simulink model "BallAndPlate_AMPC_Controller"  (R2024b)
settings: configuration reference "controller_config_MPC" (kept outside this file)
undefined symbols (not defined in the file): BallAndPlate_ss_d, TimeStep_MPC, V_refNum
libraries: mpclib x1, sharedTrackingLibrary x1
settings Model: DataDictionary=BallAndPlate_system_data.sldd  Creator=tshintai  LastModifiedBy=tshintai
settings ConfigSetRef: SourceName=controller_config_MPC

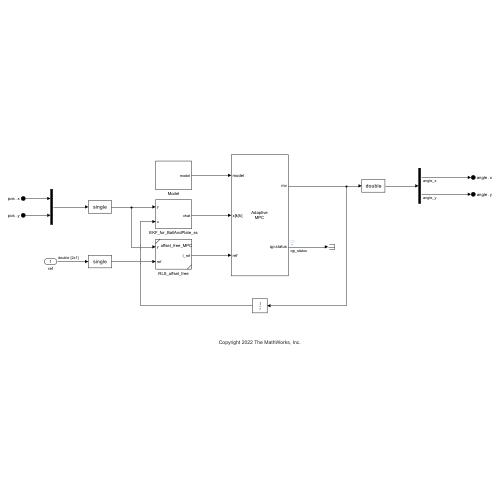
[thumbnail: Simulink's stored preview of the top-level diagram]
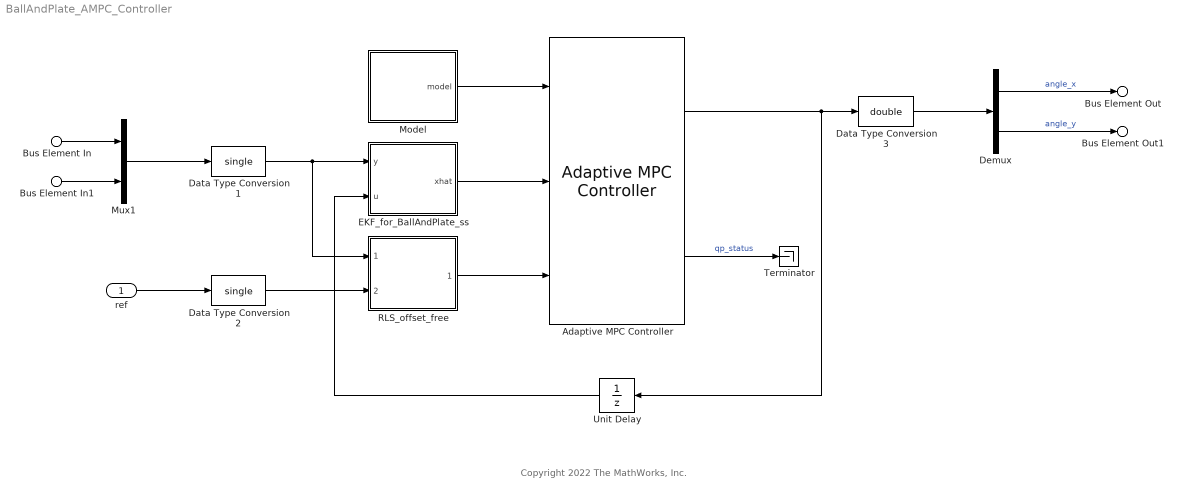
== system BallAndPlate_AMPC_Controller ==
  note: Copyright 2022 The MathWorks, Inc.
  ref : Inport  OutDataTypeStr=double  PortDimensions=[2, V_refNum]
  Bus Element In : Inport  Port=2  PortName=pos  Element=x
  Bus Element In1 : Inport  Port=2  PortName=pos  Element=y
  Adaptive MPC Controller : mpclib/Adaptive MPC Controller  SCDEnableBlockLinearizationSpecification=on  mpcobj=mpcObj  enable_value=0  updateMPCinCallerWorkspace=on  md_inport=off  mv_inport=off  uref_inport=off  return_cost=off  return_mvseq=off  return_qpstatus=on  return_xseq=off  return_state=off  return_ovseq=off  state_inport=on  isltv_plant=off  umin_inport=off  umax_inport=off  ymin_inport=off  ymax_inport=off  cc_inport=off  ywt_inport=off  uwt_inport=off  duwt_inport=off  rhoeps_inport=off  pm_inport=off  MaximumP=10  HorizonChoice=FixedHorizon  BlockDataType=single  SampleTimeInherited=off  switch_inport=off
  Data Type Conversion1 : DataTypeConversion  OutDataTypeStr=single  SaturateOnIntegerOverflow=off  RndMeth=Floor
  Data Type Conversion2 : DataTypeConversion  OutDataTypeStr=single  SaturateOnIntegerOverflow=off  RndMeth=Floor
  Data Type Conversion3 : DataTypeConversion  OutDataTypeStr=double  SaturateOnIntegerOverflow=off  RndMeth=Floor
  Demux : Demux  Outputs=2
  EKF_for_BallAndPlate_ss : Subsystem
  Model : Subsystem
  Mux1 : Mux  Inputs=2
  RLS_offset_free : Subsystem  ReferencedSubsystem=offset_free_MPC
  Terminator : Terminator
  Unit Delay : UnitDelay  SampleTime=-1  HasFrameUpgradeWarning=on
  Bus Element Out : Outport  PortName=angle  Element=x
  Bus Element Out1 : Outport  PortName=angle  Element=y
  wires:
  Bus Element In/1 -> Mux1/1
  Bus Element In1/1 -> Mux1/2
  Adaptive MPC Controller/2 -> Terminator/1  "qp_status"
  Data Type Conversion2/1 -> RLS_offset_free/2
  Model/1(model) -> Adaptive MPC Controller/1
  Adaptive MPC Controller/1 -> Data Type Conversion3/1, Unit Delay/1
  EKF_for_BallAndPlate_ss/1(xhat) -> Adaptive MPC Controller/2
  Unit Delay/1 -> EKF_for_BallAndPlate_ss/2(u)
  Data Type Conversion1/1 -> RLS_offset_free/1, EKF_for_BallAndPlate_ss/1(y)
  Data Type Conversion3/1 -> Demux/1
  Mux1/1 -> Data Type Conversion1/1
  Demux/1 -> Bus Element Out/1  "angle_x"
  Demux/2 -> Bus Element Out1/1  "angle_y"
  ref/1 -> Data Type Conversion2/1
  RLS_offset_free/1 -> Adaptive MPC Controller/3

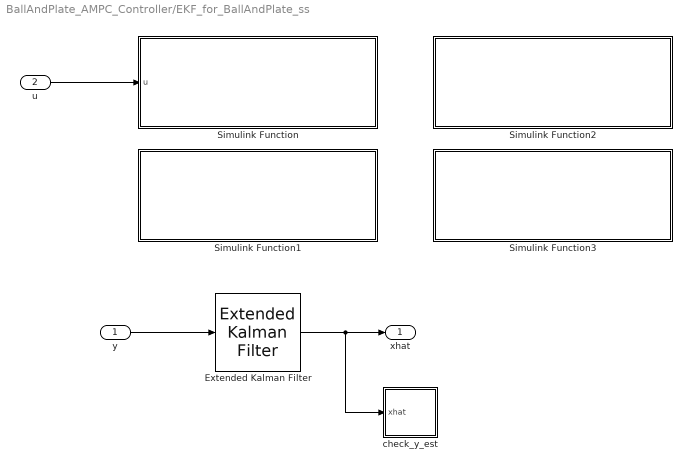
== system BallAndPlate_AMPC_Controller/EKF_for_BallAndPlate_ss ==
  y : Inport
  u : Inport  Port=2
  Extended Kalman Filter : sharedTrackingLibrary/Extended Kalman Filter  StateTransitionFcn=EKF_BAP_State_function  HasStateTransitionJacobianFcn=on  StateTransitionJacobianFcn=EKF_BAP_State_Jacobian  HasAdditiveProcessNoise=Additive  ProcessNoise=EKF_Q  HasTimeVaryingProcessNoise=off  HasStateTransitionFcnExtraArgument=0  InitialState=EKF_x_init  InitialStateCovariance=EKF_P_init  MeasurementFcn1=EKF_BAP_Measurement_function  HasMeasurementJacobianFcn1=on  MeasurementJacobianFcn1=EKF_BAP_Measurement_Jacobian  HasMeasurementEnablePort1=off  HasAdditiveMeasurementNoise1=Additive  MeasurementNoise1=EKF_R  HasTimeVaryingMeasurementNoise1=off  HasMeasurementFcnExtraArgument1=0  HasMeasurementWrapping1=off  MeasurementFcn2=myMeasurementFcn  HasMeasurementJacobianFcn2=off  HasMeasurementEnablePort2=off  HasAdditiveMeasurementNoise2=Additive  MeasurementNoise2=1  HasTimeVaryingMeasurementNoise2=off  HasMeasurementFcnExtraArgument2=0  HasMeasurementWrapping2=off  MeasurementFcn3=myMeasurementFcn  HasMeasurementJacobianFcn3=off  HasMeasurementEnablePort3=off  HasAdditiveMeasurementNoise3=Additive  MeasurementNoise3=1  HasTimeVaryingMeasurementNoise3=off  HasMeasurementFcnExtraArgument3=0  HasMeasurementWrapping3=off  MeasurementFcn4=myMeasurementFcn  HasMeasurementJacobianFcn4=off  HasMeasurementEnablePort4=off  HasAdditiveMeasurementNoise4=Additive  MeasurementNoise4=1  HasTimeVaryingMeasurementNoise4=off  HasMeasurementFcnExtraArgument4=0  HasMeasurementWrapping4=off  MeasurementFcn5=myMeasurementFcn  HasMeasurementJacobianFcn5=off  HasMeasurementEnablePort5=off  HasAdditiveMeasurementNoise5=Additive  MeasurementNoise5=1  HasTimeVaryingMeasurementNoise5=off  HasMeasurementFcnExtraArgument5=0  HasMeasurementWrapping5=off  EnableMultirate=off  StateTransitionFcnSampleTime=1  MeasurementFcn1SampleTime=1  MeasurementFcn2SampleTime=1  MeasurementFcn3SampleTime=1  MeasurementFcn4SampleTime=1  MeasurementFcn5SampleTime=1  UseCurrentEstimator=on  OutputStateCovariance=off  DataType=single  SampleTime=TimeStep_MPC  NumberOfMeasurements=1
  Simulink Function : Subsystem  TreatAsAtomicUnit=on
  Simulink Function1 : Subsystem  TreatAsAtomicUnit=on
  Simulink Function2 : Subsystem  TreatAsAtomicUnit=on
  Simulink Function3 : Subsystem  TreatAsAtomicUnit=on
  check_y_est : Subsystem
  xhat : Outport
  wires:
  u/1 -> Simulink Function/1(u)
  Extended Kalman Filter/1 -> check_y_est/1(xhat), xhat/1
  y/1 -> Extended Kalman Filter/1

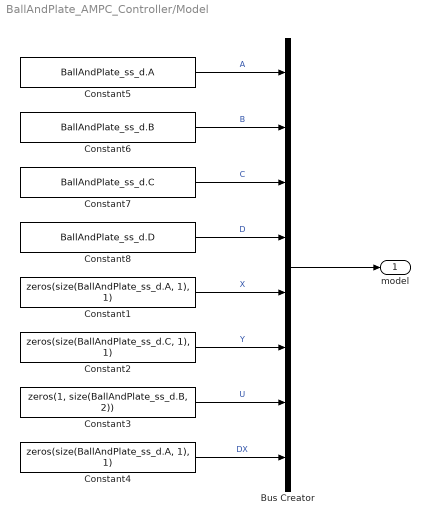
== system BallAndPlate_AMPC_Controller/Model ==
  Bus Creator : BusCreator  Inputs=8
  Constant1 : Constant  Value=zeros(size(BallAndPlate_ss_d.A, 1), 1)  VectorParams1D=off  OutDataTypeStr=single
  Constant2 : Constant  Value=zeros(size(BallAndPlate_ss_d.C, 1), 1)  VectorParams1D=off  OutDataTypeStr=single
  Constant3 : Constant  Value=zeros(1, size(BallAndPlate_ss_d.B, 2))  VectorParams1D=off  OutDataTypeStr=single
  Constant4 : Constant  Value=zeros(size(BallAndPlate_ss_d.A, 1), 1)  VectorParams1D=off  OutDataTypeStr=single
  Constant5 : Constant  Value=BallAndPlate_ss_d.A  VectorParams1D=off  OutDataTypeStr=single
  Constant6 : Constant  Value=BallAndPlate_ss_d.B  VectorParams1D=off  OutDataTypeStr=single
  Constant7 : Constant  Value=BallAndPlate_ss_d.C  VectorParams1D=off  OutDataTypeStr=single
  Constant8 : Constant  Value=BallAndPlate_ss_d.D  VectorParams1D=off  OutDataTypeStr=single
  model : Outport
  wires:
  Constant2/1 -> Bus Creator/6  "Y"
  Constant5/1 -> Bus Creator/1  "A"
  Constant6/1 -> Bus Creator/2  "B"
  Bus Creator/1 -> model/1
  Constant7/1 -> Bus Creator/3  "C"
  Constant8/1 -> Bus Creator/4  "D"
  Constant3/1 -> Bus Creator/7  "U"
  Constant4/1 -> Bus Creator/8  "DX"
  Constant1/1 -> Bus Creator/5  "X"

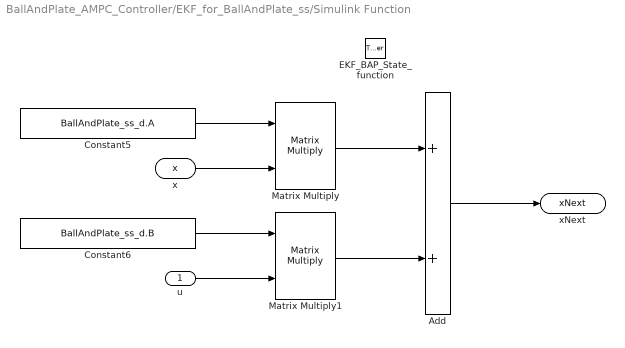
== system BallAndPlate_AMPC_Controller/EKF_for_BallAndPlate_ss/Simulink Function ==
  u : Inport
  EKF_BAP_State_function : TriggerPort  TriggerType=function-call  IsSimulinkFunction=on  FunctionName=EKF_BAP_State_function  FunctionVisibility=scoped  VariantControl=(inherit)
  Add : Sum
  Constant5 : Constant  Value=BallAndPlate_ss_d.A  VectorParams1D=off  OutDataTypeStr=single
  Constant6 : Constant  Value=BallAndPlate_ss_d.B  VectorParams1D=off  OutDataTypeStr=single
  Matrix Multiply : Product  Multiplication=Matrix(*)
  Matrix Multiply1 : Product  Multiplication=Matrix(*)
  x : ArgIn  DisableCoverage=on  OutDataTypeStr=single  PortDimensions=size(BallAndPlate_ss_d.A, 1)  ArgumentName=x
  xNext : ArgOut  DisableCoverage=on  OutDataTypeStr=single  PortDimensions=size(BallAndPlate_ss_d.A, 1)  ArgumentName=xNext
  wires:
  x/1 -> Matrix Multiply/2
  Constant5/1 -> Matrix Multiply/1
  u/1 -> Matrix Multiply1/2
  Constant6/1 -> Matrix Multiply1/1
  Matrix Multiply/1 -> Add/1
  Matrix Multiply1/1 -> Add/2
  Add/1 -> xNext/1

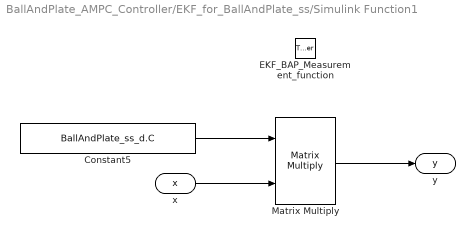
== system BallAndPlate_AMPC_Controller/EKF_for_BallAndPlate_ss/Simulink Function1 ==
  EKF_BAP_Measurement_function : TriggerPort  TriggerType=function-call  IsSimulinkFunction=on  FunctionName=EKF_BAP_Measurement_function  FunctionVisibility=scoped  VariantControl=(inherit)
  Constant5 : Constant  Value=BallAndPlate_ss_d.C  VectorParams1D=off  OutDataTypeStr=single
  Matrix Multiply : Product  Multiplication=Matrix(*)
  x : ArgIn  DisableCoverage=on  OutDataTypeStr=single  PortDimensions=size(BallAndPlate_ss_d.A, 1)  ArgumentName=x
  y : ArgOut  DisableCoverage=on  OutDataTypeStr=single  PortDimensions=size(BallAndPlate_ss_d.C, 1)  ArgumentName=y
  wires:
  Constant5/1 -> Matrix Multiply/1
  x/1 -> Matrix Multiply/2
  Matrix Multiply/1 -> y/1

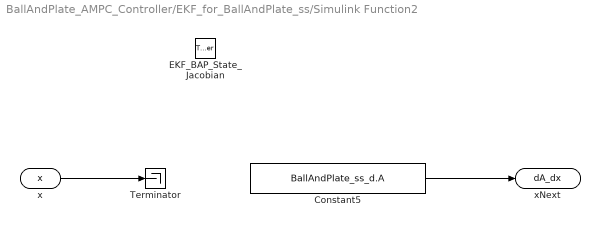
== system BallAndPlate_AMPC_Controller/EKF_for_BallAndPlate_ss/Simulink Function2 ==
  EKF_BAP_State_Jacobian : TriggerPort  TriggerType=function-call  IsSimulinkFunction=on  FunctionName=EKF_BAP_State_Jacobian  FunctionVisibility=scoped  VariantControl=(inherit)
  Constant5 : Constant  Value=BallAndPlate_ss_d.A  VectorParams1D=off  OutDataTypeStr=single
  Terminator : Terminator
  x : ArgIn  DisableCoverage=on  OutDataTypeStr=single  PortDimensions=size(BallAndPlate_ss_d.A, 1)  ArgumentName=x
  xNext : ArgOut  DisableCoverage=on  OutDataTypeStr=single  PortDimensions=size(BallAndPlate_ss_d.A)  ArgumentName=dA_dx
  wires:
  Constant5/1 -> xNext/1
  x/1 -> Terminator/1

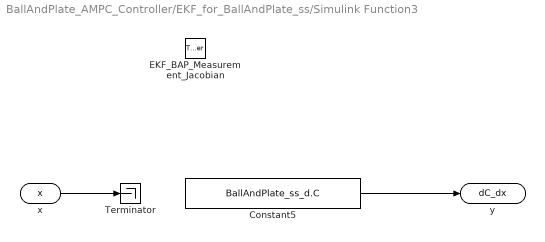
== system BallAndPlate_AMPC_Controller/EKF_for_BallAndPlate_ss/Simulink Function3 ==
  EKF_BAP_Measurement_Jacobian : TriggerPort  TriggerType=function-call  IsSimulinkFunction=on  FunctionName=EKF_BAP_Measurement_Jacobian  FunctionVisibility=scoped  VariantControl=(inherit)
  Constant5 : Constant  Value=BallAndPlate_ss_d.C  VectorParams1D=off  OutDataTypeStr=single
  Terminator : Terminator
  x : ArgIn  DisableCoverage=on  OutDataTypeStr=single  PortDimensions=size(BallAndPlate_ss_d.A, 1)  ArgumentName=x
  y : ArgOut  DisableCoverage=on  OutDataTypeStr=single  PortDimensions=size(BallAndPlate_ss_d.C)  ArgumentName=dC_dx
  wires:
  Constant5/1 -> y/1
  x/1 -> Terminator/1

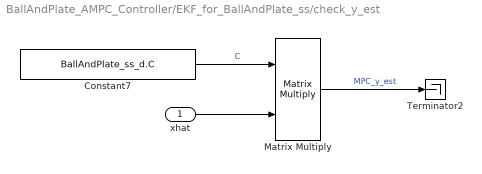
== system BallAndPlate_AMPC_Controller/EKF_for_BallAndPlate_ss/check_y_est ==
  xhat : Inport
  Constant7 : Constant  Value=BallAndPlate_ss_d.C  VectorParams1D=off  OutDataTypeStr=single
  Matrix Multiply : Product  Multiplication=Matrix(*)
  Terminator2 : Terminator
  wires:
  Matrix Multiply/1 -> Terminator2/1  "MPC_y_est"
  Constant7/1 -> Matrix Multiply/1  "C"
  xhat/1 -> Matrix Multiply/2
